simulink model "duffing_simulation_ss"  (R2018a)
settings: Solver=ode23  StartTime=0.0  StopTime=100  RelTol=1e-3
values from neighbouring files (symbols this model uses):
  zeta = 1/(2*Q)    (= 0.005)    [sim_run.m]
undefined symbols (not defined in the file or in its folder): D, N, R
settings Model: Creator=Shay  LastModifiedBy=Shay

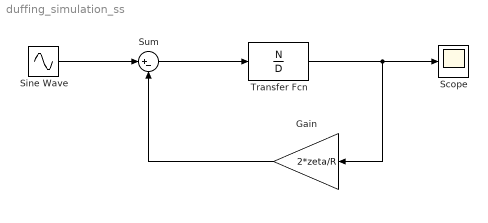
== system duffing_simulation_ss ==
  Gain : Gain  Gain=2*zeta/R
  Scope : Scope
  Sine Wave : Sin  Amplitude=2  SampleTime=1
  Sum : Sum  Inputs=|+-
  Transfer Fcn : TransferFcn  Numerator=N  Denominator=D
  wires:
  Sine Wave/1 -> Sum/1
  Transfer Fcn/1 -> Gain/1, Scope/1
  Sum/1 -> Transfer Fcn/1
  Gain/1 -> Sum/2
